simulink model "droneSim"  (R2021a)
settings: Solver=ode4  StartTime=0.0  StopTime=10.0  FixedStep=1/simVars.freq  RelTol=1e-3
undefined symbols (not defined in the file): sigbuilder_block, simVars
libraries: simulink x1
settings Model: Creator=Matthias  LastModifiedBy=root
settings SolverCC: AlgebraicLoopSolver=TrustRegion
settings DataIOCC: ReturnWorkspaceOutputs=off
settings DebuggingCC: SFMachineParentedDataDiag=warning  ArithmeticOperatorsInVariantConditions=warning
settings SFSimCC: CustomCodeUndefinedFunction=UseInterfaceOnly

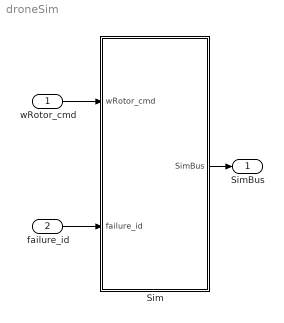
== system droneSim ==
  wRotor_cmd : Inport
  failure_id : Inport  Port=2
  Sim : Subsystem
  SimBus : Outport  OutDataTypeStr=Bus: simBus  VectorParamsAs1DForOutWhenUnconnected=off
  wires:
  wRotor_cmd/1 -> Sim/1(wRotor_cmd)
  Sim/1(SimBus) -> SimBus/1
  failure_id/1 -> Sim/2(failure_id)

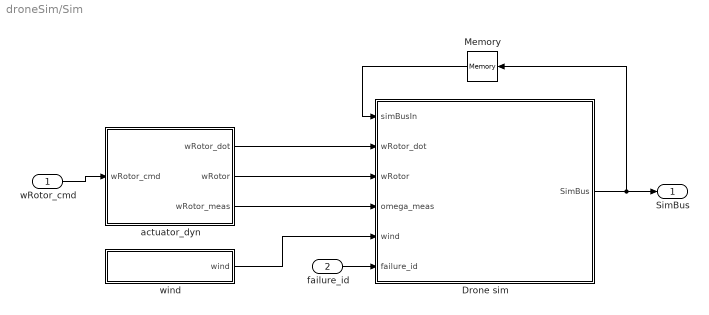
== system droneSim/Sim ==
  wRotor_cmd : Inport
  failure_id : Inport  Port=2
  Drone sim : Subsystem
  Memory : Memory
  actuator_dyn : Subsystem
  wind : Subsystem
  SimBus : Outport  OutDataTypeStr=Bus: simBus  VectorParamsAs1DForOutWhenUnconnected=off
  wires:
  wRotor_cmd/1 -> actuator_dyn/1(wRotor_cmd)
  actuator_dyn/1(wRotor_dot) -> Drone sim/2(wRotor_dot)
  actuator_dyn/2(wRotor) -> Drone sim/3(wRotor)
  wind/1(wind) -> Drone sim/5(wind)
  Drone sim/1(SimBus) -> Memory/1, SimBus/1
  Memory/1 -> Drone sim/1(simBusIn)
  actuator_dyn/3(wRotor_meas) -> Drone sim/4(omega_meas)
  failure_id/1 -> Drone sim/6(failure_id)

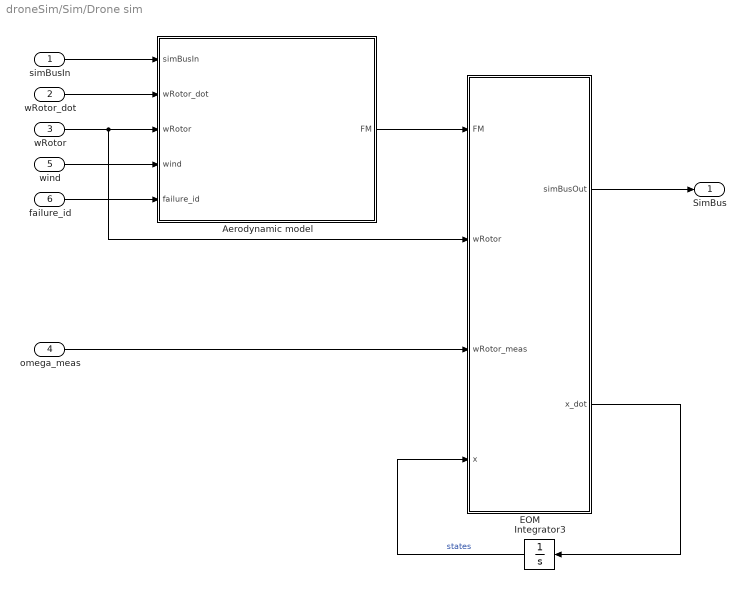
== system droneSim/Sim/Drone sim ==
  simBusIn : Inport
  wRotor_dot : Inport  Port=2
  wRotor : Inport  Port=3
  omega_meas : Inport  Port=4
  wind : Inport  Port=5
  failure_id : Inport  Port=6
  Aerodynamic model : MATLAB Function  TreatAsAtomicUnit=on
  EOM : MATLAB Function  TreatAsAtomicUnit=on
  Integrator3 : Integrator  InitialCondition=[simVars.pos0,simVars.vel0,simVars.q0,simVars.omega0,simVars.att0]
  SimBus : Outport  VectorParamsAs1DForOutWhenUnconnected=off
  wires:
  wRotor/1 -> EOM/2(wRotor), Aerodynamic model/3(wRotor)
  simBusIn/1 -> Aerodynamic model/1(simBusIn)
  wRotor_dot/1 -> Aerodynamic model/2(wRotor_dot)
  wind/1 -> Aerodynamic model/4(wind)
  omega_meas/1 -> EOM/3(wRotor_meas)
  EOM/2(x_dot) -> Integrator3/1
  Integrator3/1 -> EOM/4(x)  "states"
  EOM/1(simBusOut) -> SimBus/1
  Aerodynamic model/1(FM) -> EOM/1(FM)
  failure_id/1 -> Aerodynamic model/5(failure_id)

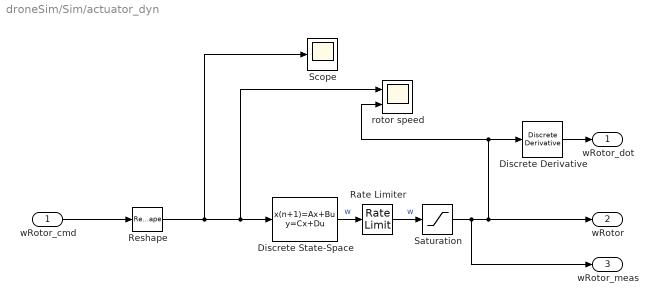
== system droneSim/Sim/actuator_dyn ==
  wRotor_cmd : Inport
  Discrete Derivative : simulink/Discrete/Discrete Derivative  gainval=1.0  ICPrevScaledInput=0.0  OutMin=[]  OutMax=[]  OutDataType=fixdt(1, 16)  OutScaling=2^-10  DoSatur=off
  Discrete State-Space : DiscreteStateSpace  A=(1-1/simVars.actuator.t_w*1/simVars.freq)*eye(4)  B=1/simVars.actuator.t_w*1/simVars.freq*eye(4)  C=eye(4)  D=zeros(4)  InitialCondition=simVars.actuator.w0  SampleTime=-1
  Rate Limiter : RateLimiter  RisingSlewLimit=simVars.actuator.rateRise  FallingSlewLimit=simVars.actuator.rateFall  SampleTimeMode=inherited  InitialCondition=simVars.actuator.w0  LinearizeAsGain=off
  Reshape : Reshape
  Saturation : Saturate  UpperLimit=simVars.actuator.wMax  LowerLimit=simVars.actuator.wMin
  Scope : Scope
  rotor speed : Scope  NumInputPorts=2
  wRotor_dot : Outport  VectorParamsAs1DForOutWhenUnconnected=off
  wRotor : Outport  Port=2  VectorParamsAs1DForOutWhenUnconnected=off
  wRotor_meas : Outport  Port=3  VectorParamsAs1DForOutWhenUnconnected=off
  wires:
  wRotor_cmd/1 -> Reshape/1
  Rate Limiter/1 -> Saturation/1  "w"
  Discrete Derivative/1 -> wRotor_dot/1
  Reshape/1 -> Scope/1, Discrete State-Space/1, rotor speed/1
  Saturation/1 -> wRotor_meas/1, Discrete Derivative/1, rotor speed/2, wRotor/1
  Discrete State-Space/1 -> Rate Limiter/1  "w"

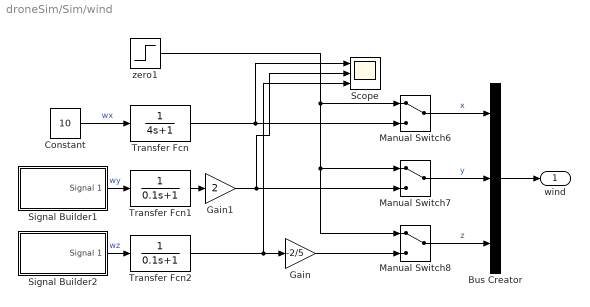
== system droneSim/Sim/wind ==
  Bus Creator : BusCreator  Inputs=3  OutDataTypeStr=Bus: windBus
  Constant : Constant  Value=10
  Gain : Gain  Gain=-2/5
  Gain1 : Gain  Gain=2
  Manual Switch6 : ManualSwitch
  Manual Switch7 : ManualSwitch
  Manual Switch8 : ManualSwitch
  Scope : Scope  NumInputPorts=3
  Signal Builder1 : Subsystem  Tag=STV Subsys  LoadFcn=sigbuilder_block('load');  StartFcn=sigbuilder_block('start');  StopFcn=sigbuilder_block('stop');  ClipboardFcn=sigbuilder_block('clipboard');  mask(Sigbuilder block){tuvar=[0:10]}
      mask help: Simulink:masks:SigbuilderBlock_MD
      mask init:
      | if ~strcmp(get_param(bdroot(gcbh),'SimulationStatus'),'stopped') tuvar = sigbuilder_block('maskInit'); end
      settings: CopyFcn=sigbuilder_block('copy');  DeleteFcn=sigbuilder_block('delete');  ModelCloseFcn=sigbuilder_block('modelClose');  PreSaveFcn=sigbuilder_block('preSave');  PauseFcn=sigbuilder_block('pause');  ContinueFcn=sigbuilder_block('continue');  NameChangeFcn=sigbuilder_block('namechange');  OpenFcn=sigbuilder_block('open',[196.5 289.5 550.5 399.75 ]);  CloseFcn=sigbuilder_block('close');
      mask Display: plot(0, 0, 100, 100,[2, 2, 32, 32, 2], [68, 8, 8, 68, 68],[32, 2], [38, 38], [32, 19, 2],[53, 60, 44], [32, 17, 17, 2],[16, 16, 31, 31]);txt = getActiveGroup(gcbh);text(2, 100, txt,'verticalAlignment', 'top');
  Signal Builder2 : Subsystem  Tag=STV Subsys  LoadFcn=sigbuilder_block('load');  StartFcn=sigbuilder_block('start');  StopFcn=sigbuilder_block('stop');  ClipboardFcn=sigbuilder_block('clipboard');  mask(Sigbuilder block){tuvar=[0:10]}
      mask help: Simulink:masks:SigbuilderBlock_MD
      mask init:
      | if ~strcmp(get_param(bdroot(gcbh),'SimulationStatus'),'stopped') tuvar = sigbuilder_block('maskInit'); end
      settings: CopyFcn=sigbuilder_block('copy');  DeleteFcn=sigbuilder_block('delete');  ModelCloseFcn=sigbuilder_block('modelClose');  PreSaveFcn=sigbuilder_block('preSave');  PauseFcn=sigbuilder_block('pause');  ContinueFcn=sigbuilder_block('continue');  NameChangeFcn=sigbuilder_block('namechange');  OpenFcn=sigbuilder_block('open',[229.5 273.75 550.5 399.75 ]);  CloseFcn=sigbuilder_block('close');
      mask Display: plot(0, 0, 100, 100,[2, 2, 32, 32, 2], [68, 8, 8, 68, 68],[32, 2], [38, 38], [32, 19, 2],[53, 60, 44], [32, 17, 17, 2],[16, 16, 31, 31]);txt = getActiveGroup(gcbh);text(2, 100, txt,'verticalAlignment', 'top');
  Transfer Fcn : TransferFcn  Denominator=[4 1]
  Transfer Fcn1 : TransferFcn  Denominator=[0.1 1]
  Transfer Fcn2 : TransferFcn  Denominator=[0.1 1]
  zero1 : Step  Time=5  After=0  SampleTime=0
  wind : Outport  VectorParamsAs1DForOutWhenUnconnected=off
  wires:
  Manual Switch7/1 -> Bus Creator/2  "y"
  Manual Switch6/1 -> Bus Creator/1  "x"
  Signal Builder2/1(Signal 1) -> Transfer Fcn2/1  "wz"
  zero1/1 -> Manual Switch8/1, Manual Switch7/1, Manual Switch6/1
  Signal Builder1/1(Signal 1) -> Transfer Fcn1/1  "wy"
  Manual Switch8/1 -> Bus Creator/3  "z"
  Constant/1 -> Transfer Fcn/1  "wx"
  Transfer Fcn2/1 -> Scope/3, Gain/1
  Transfer Fcn1/1 -> Gain1/1
  Gain/1 -> Manual Switch8/2
  Gain1/1 -> Scope/2, Manual Switch7/2
  Transfer Fcn/1 -> Scope/1, Manual Switch6/2
  Bus Creator/1 -> wind/1

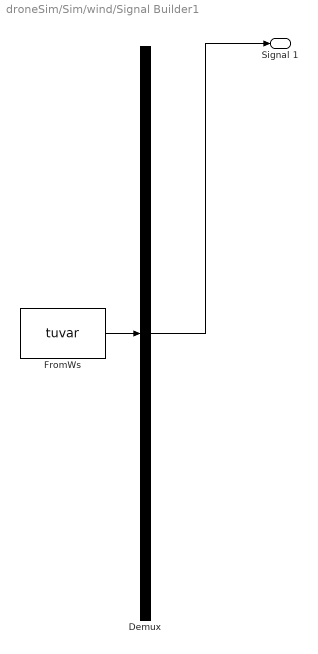
== system droneSim/Sim/wind/Signal Builder1 ==
  Demux : Demux  Tag=STV Demux  Outputs=1
      settings: DisplayOption=none
  FromWs : FromWorkspace  Tag=STV FromWs  VariableName=tuvar
      SigBuilderData=|
      | common.afterFinalStr = 'Extrapolate'
      | common.sampleTime = 0
      | dataSet.timeRange = [0 20]
      | dataSet.name = 'Group 1'
      | sbobj.Groups.Name = 'Group 1'
      | sbobj.Groups.Signals.Name = 'Signal 1'
      | sbobj.Groups.Signals.XData = [0 4 4 10 10 18 18 20]
      | sbobj.Groups.Signals.YData = [0 0 2 2 -2 -2 0 0.01]
      | sbobj.Groups.TimeRange = [0 20]
  Signal 1 : Outport  Tag=STV Outport  VectorParamsAs1DForOutWhenUnconnected=off
  wires:
  FromWs/1 -> Demux/1
  Demux/1 -> Signal 1/1

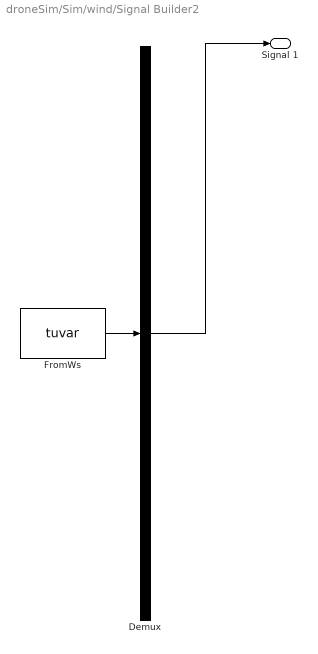
== system droneSim/Sim/wind/Signal Builder2 ==
  Demux : Demux  Tag=STV Demux  Outputs=1
      settings: DisplayOption=none
  FromWs : FromWorkspace  Tag=STV FromWs  VariableName=tuvar
      SigBuilderData=|
      | common.afterFinalStr = 'Extrapolate'
      | common.sampleTime = 0
      | dataSet.timeRange = [0 20]
      | dataSet.name = 'Group 1'
      | sbobj.Groups.Name = 'Group 1'
      | sbobj.Groups.Signals.Name = 'Signal 1'
      | sbobj.Groups.Signals.XData = [0 3 3 8 8 12 12 16 20]
      | sbobj.Groups.Signals.YData = [0 0 5 5.00666666667 5 5 5.01333333333 5 5]
      | sbobj.Groups.TimeRange = [0 20]
  Signal 1 : Outport  Tag=STV Outport  VectorParamsAs1DForOutWhenUnconnected=off
  wires:
  FromWs/1 -> Demux/1
  Demux/1 -> Signal 1/1

== matlab function droneSim/Sim/Drone sim/EOM ==
  settings: updateMethod=DISCRETE
  data: simBusOut output Bus: simBus; FM input; wRotor input; wRotor_meas input; x input; simVars parameter; x_dot output
function [simBusOut,x_dot] = EOM(FM, wRotor, wRotor_meas, x, simVars)
[simBusOut, x_dot] = EOMQuat(FM,wRotor,wRotor_meas,x,simVars);

== matlab function droneSim/Sim/Drone sim/Aerodynamic model ==
  settings: updateMethod=DISCRETE
  data: simBusIn input Bus: simBus; FM output Bus: FMBus; wRotor_dot input; wRotor input; wind input Bus: windBus; simVars parameter; failure_id input
function FM = aeroModel(simBusIn, wRotor_dot, wRotor, wind, simVars, failure_id)
    FM = aeroModel(simBusIn, wRotor_dot, wRotor, wind, simVars, failure_id);
end
